simulink model "CoVeh"  (R2018a)
settings: configuration reference "cs_ert" (kept outside this file)
settings Model: DataDictionary=CoVeh.sldd  Creator=zhoutinglin  LastModifiedBy=zhoutinglin

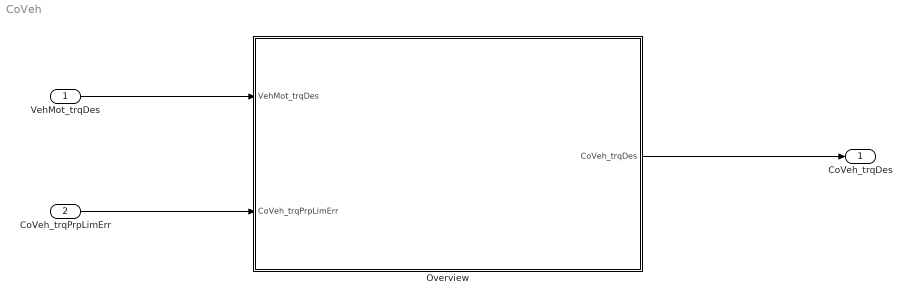
== system CoVeh ==
  VehMot_trqDes : Inport
  CoVeh_trqPrpLimErr : Inport  Port=2
  Overview : Subsystem
  CoVeh_trqDes : Outport
  wires:
  VehMot_trqDes/1 -> Overview/1(VehMot_trqDes)
  CoVeh_trqPrpLimErr/1 -> Overview/2(CoVeh_trqPrpLimErr)
  Overview/1(CoVeh_trqDes) -> CoVeh_trqDes/1

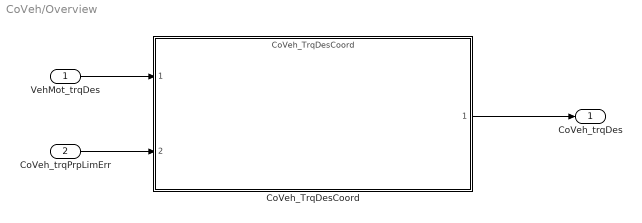
== system CoVeh/Overview ==
  VehMot_trqDes : Inport
  CoVeh_trqPrpLimErr : Inport  Port=2
  CoVeh_TrqDesCoord : ModelReference  ModelNameDialog=CoVeh_TrqDesCoord  SimulationMode=Normal  ModelReferenceVersion=1.49
  CoVeh_trqDes : Outport
  wires:
  VehMot_trqDes/1 -> CoVeh_TrqDesCoord/1
  CoVeh_trqPrpLimErr/1 -> CoVeh_TrqDesCoord/2
  CoVeh_TrqDesCoord/1 -> CoVeh_trqDes/1
